simulink model "PiCube_task"  (Simulink 7.5)
libraries: mathlib x13, speclib x3
settings Model: Creator=jsobota  LastModifiedBy=jsobota  ExtModeTrigMode=oneshot  ExtModeArmWhenConnect=off

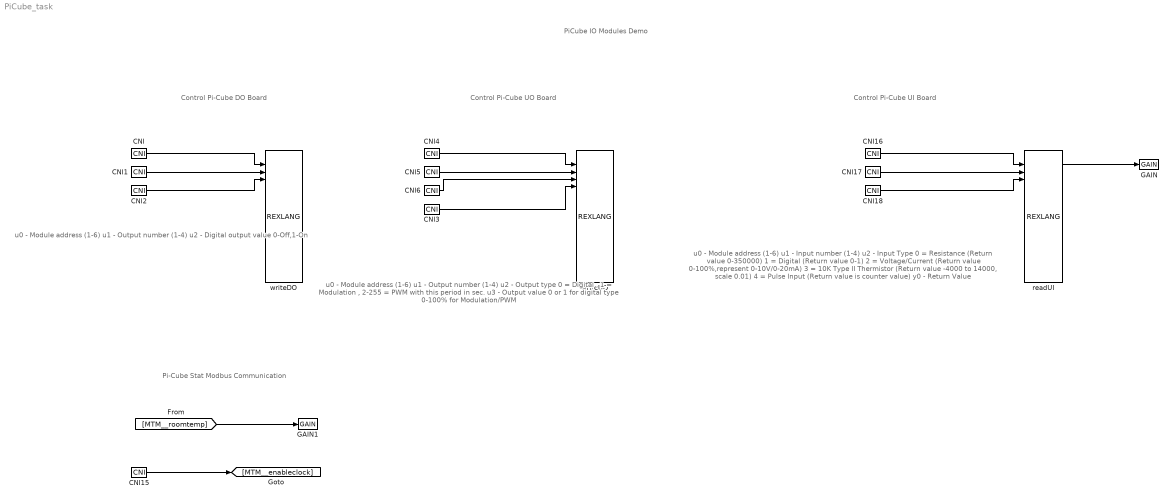
== system PiCube_task ==
  note: Control Pi-Cube DO Board
  note: u0 - Module address (1-6)
      | u1 - Output number (1-4)
      | u2  - Digital output value 0-Off,1-On
  note: Control Pi-Cube UO Board
  note: u0 - Module address (1-6)
      | u1 - Output number (1-4)
      | u2 - Output type
      |             0 = Digital ,
      |             1 = Modulation ,
      |             2-255 = PWM with this period in sec.
      | u3 - Output value
      |             0 or 1 for digital type
      |             0-100% for Modulation/PWM
  note: PiCube IO Modules Demo
  note: u0 - Module address (1-6)
      | u1 - Input number (1-4)
      | u2  - Input Type
      |             0 = Resistance (Return value 0-350000)
      |             1 = Digital (Return value 0-1)
      |             2 = Voltage/Current (Return value 0-100%,represent 0-10V/0-20mA)
      |             3 = 10K Type II Thermistor (Return value -4000 to 14000, scale 0.01)
      |             4 = Pulse Input (Return value is counter value)
      |
      | y0 - Return Value
  note: Pi-Cube Stat Modbus Communication
  note: Control Pi-Cube UI Board
  CNI : mathlib/CNI  icn=5
  CNI{1..2,5,15..17} (6 alike) : mathlib/CNI  icn=1
  CNI18 : mathlib/CNI  icn=3
  CNI3 : mathlib/CNI  icn=0
  CNI4 : mathlib/CNI  icn=4
  CNI6 : mathlib/CNI  icn=0
  GAIN : mathlib/GAIN  k=0.01
  GAIN1 : mathlib/GAIN  k=0.1
  readUI : speclib/REXLANG  SystemSampleTime=-1  tab_matlab=BASIC  srcname=readUI.c  srctype=1: STL  stack=0  debug=1: No check  p0=0  p1=0  p2=0  p3=0  p4=0  p5=0  p6=0  p7=0  p8=0  p9=0  p10=0  p11=0  p12=0  p13=0  p14=0  p15=0  fname=/dev/i2c-1
  writeDO : speclib/REXLANG  SystemSampleTime=-1  tab_matlab=BASIC  srcname=writeDO.c  srctype=1: STL  stack=0  debug=1: No check  p0=0  p1=0  p2=0  p3=0  p4=0  p5=0  p6=0  p7=0  p8=0  p9=0  p10=0  p11=0  p12=0  p13=0  p14=0  p15=0  fname=/dev/i2c-1
  writeUO : speclib/REXLANG  SystemSampleTime=-1  tab_matlab=BASIC  srcname=writeUO.c  srctype=1: STL  stack=0  debug=1: No check  p0=0  p1=0  p2=0  p3=0  p4=0  p5=0  p6=0  p7=0  p8=0  p9=0  p10=0  p11=0  p12=0  p13=0  p14=0  p15=0  fname=/dev/i2c-1
  wires:
  CNI/1 -> writeDO/2
  CNI1/1 -> writeDO/3
  CNI15/1 -> [MTM__enableclock]
  CNI16/1 -> readUI/2
  CNI17/1 -> readUI/3
  CNI18/1 -> readUI/4
  CNI2/1 -> writeDO/4
  CNI3/1 -> writeUO/5
  CNI4/1 -> writeUO/2
  CNI5/1 -> writeUO/3
  CNI6/1 -> writeUO/4
  [MTM__roomtemp] -> GAIN1/1
  readUI/2 -> GAIN/1
